simulink model "Exam_Observer_Controller"  (R2022b)
settings: Solver=VariableStepAuto  StartTime=0.0  StopTime=10.0  RelTol=1e-3
values from neighbouring files (symbols this model uses):
  A = [0 1;-20 -3]    [Code.m]
  B = [0;1]    [Code.m]
  C = [1 0]    [Code.m]
  D = [0 0]    [Code.m]
  K = acker(A, B, J)    [Code.m]
settings Model: Creator=adlercohen  LastModifiedBy=adlercohen

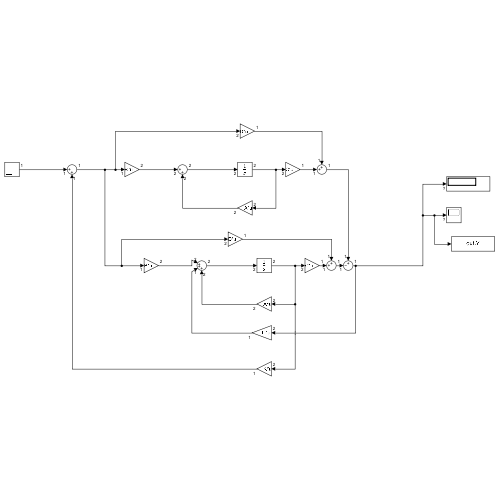
[thumbnail: Simulink's stored preview of the top-level diagram]
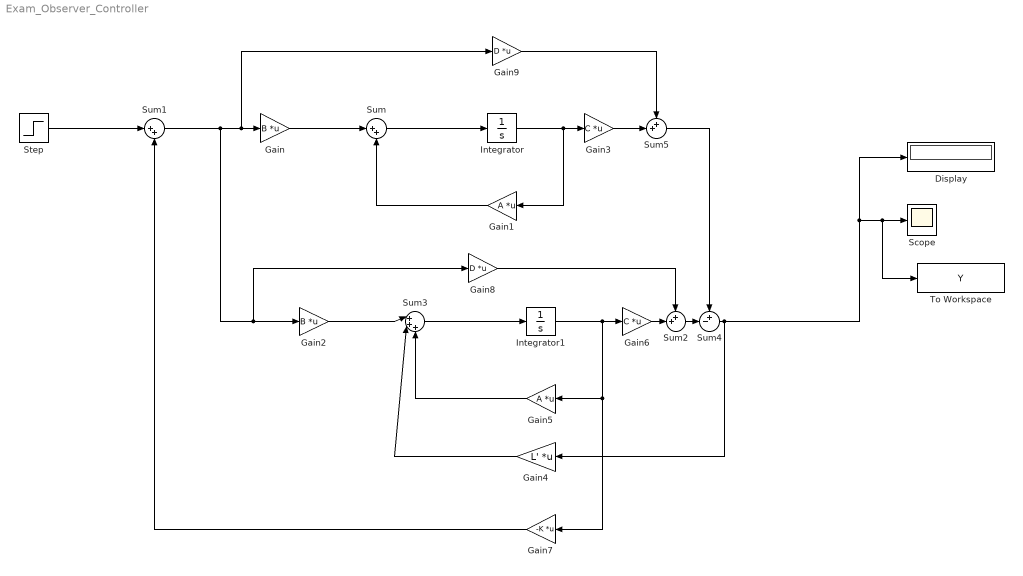
== system Exam_Observer_Controller ==
  Display : Display
  Gain : Gain  Gain=B  Multiplication=Matrix(K*u)
  Gain1 : Gain  Gain=A  Multiplication=Matrix(K*u)
  Gain2 : Gain  Gain=B  Multiplication=Matrix(K*u)
  Gain3 : Gain  Gain=C  Multiplication=Matrix(K*u)
  Gain4 : Gain  Gain=L'  Multiplication=Matrix(K*u)
  Gain5 : Gain  Gain=A  Multiplication=Matrix(K*u)
  Gain6 : Gain  Gain=C  Multiplication=Matrix(K*u)
  Gain7 : Gain  Gain=-K  Multiplication=Matrix(K*u)
  Gain8 : Gain  Gain=D  Multiplication=Matrix(K*u)
  Gain9 : Gain  Gain=D  Multiplication=Matrix(K*u)
  Integrator : Integrator
  Integrator1 : Integrator
  Scope : Scope
  Step : Step  Time=0  SampleTime=0
  Sum : Sum  Inputs=|++
  Sum1 : Sum  Inputs=|++
  Sum2 : Sum  Inputs=++|
  Sum3 : Sum  Inputs=|+++
  Sum4 : Sum  Inputs=+-|
  Sum5 : Sum  Inputs=++|
  To Workspace : ToWorkspace  VariableName=Y  SampleTime=-1
  wires:
  Sum/1 -> Integrator/1
  Step/1 -> Sum1/1
  Integrator/1 -> Gain1/1, Gain3/1
  Gain/1 -> Sum/1
  Gain1/1 -> Sum/2
  Gain5/1 -> Sum3/3
  Gain2/1 -> Sum3/1
  Sum1/1 -> Gain8/1, Gain2/1, Gain9/1, Gain/1
  Sum3/1 -> Integrator1/1
  Integrator1/1 -> Gain7/1, Gain5/1, Gain6/1
  Sum4/1 -> Gain4/1, Display/1, To Workspace/1, Scope/1
  Gain4/1 -> Sum3/2
  Gain7/1 -> Sum1/2
  Gain6/1 -> Sum2/2
  Sum2/1 -> Sum4/2
  Gain8/1 -> Sum2/1
  Gain9/1 -> Sum5/1
  Gain3/1 -> Sum5/2
  Sum5/1 -> Sum4/1
